simulink model "ES_butterfinger"  (R2017b)
settings: Solver=ode5  StartTime=0.0  StopTime=t_end  FixedStep=dt  RelTol=1e-3
values from neighbouring files (symbols this model uses):
  decimal_year = year + (DOY./365) + (hour./(365.*24)) + (minute./(365.*24.*60)) + (second./(365.*24.*3600))    [Sim_Starter.m]
  DOY = make_doy(year,month,day)    [Sim_Starter.m]    (also in make_doy.m = day + month_doy)
  Ib = [50 0 0; 0 50 0; 0 0 25]    [Sim_Starter.m]
  IC = [r_ECI_i; v_ECI_i; q_i; w_i]    [Sim_Starter.m]
  msc = 50    [Sim_Starter.m]
  sc_area = [1; 1; 1]    [Sim_Starter.m]
  sc_cop = [0; 0; 0]    [Sim_Starter.m]
  year = 2017    [Sim_Starter.m]
undefined symbols (not defined in the file or in its folder): DiscIntNeverNeededParam, Earth, IAU, WGS84
libraries: aerolibtransform2 x3, sharedtransform x3, aerolibatmos2 x1, aerolibgravity2 x1
settings Model: Creator=Mitchel  LastModifiedBy=Mitchel

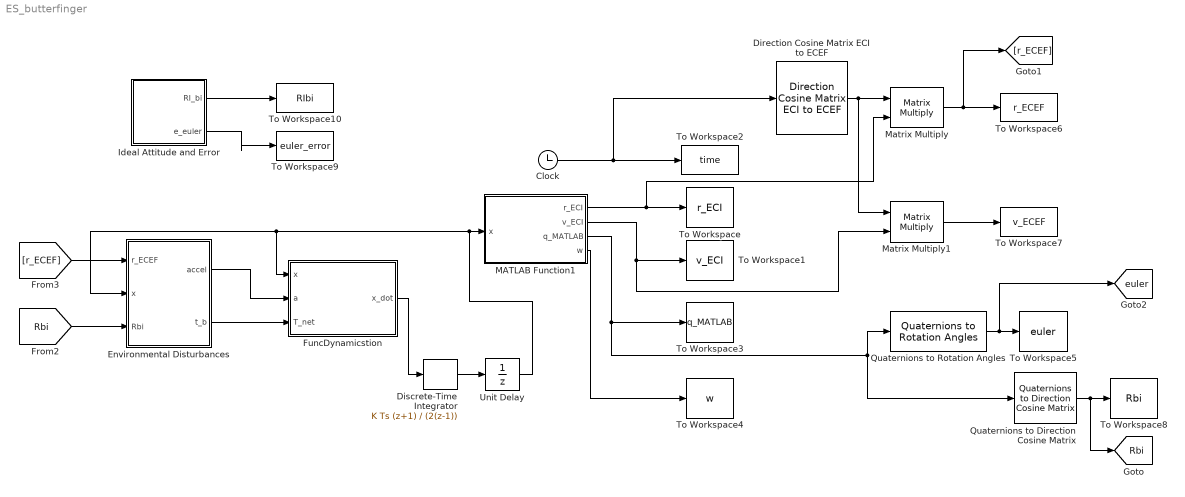
== system ES_butterfinger ==
  Clock : Clock
  Direction Cosine Matrix ECI to ECEF : aerolibtransform2/Direction Cosine Matrix ECI to ECEF  red=IAU-2000/2006  year=year  month=November  day=20  hour=hour  min=minute  sec=second  deltaT=Sec  errorflag=Error  extraparamflag=off
      settings: AttributesFormatString=%<red>  SourceProductName=Aerospace Blockset  SourceProductBaseCode=AE
  Discrete-Time Integrator : DiscreteIntegrator  IntegratorMethod=Integration: Trapezoidal  InitialCondition=IC  InitialConditionSetting=State (most efficient)  SampleTime=-1  ICPrevOutput=DiscIntNeverNeededParam  ICPrevScaledInput=DiscIntNeverNeededParam
  Environmental Disturbances : Subsystem
  FuncDynamicstion : MATLAB Function  TreatAsAtomicUnit=on
  Ideal Attitude and Error : Subsystem
  MATLAB Function1 : MATLAB Function  TreatAsAtomicUnit=on
  Matrix Multiply : Product  Multiplication=Matrix(*)
  Matrix Multiply1 : Product  Multiplication=Matrix(*)
  Quaternions to Direction Cosine Matrix : sharedtransform/Quaternions to  Direction Cosine Matrix
      settings: SourceProductName=Aerospace Blockset  SourceProductBaseCode=AE
  Quaternions to Rotation Angles : sharedtransform/Quaternions to Rotation Angles  rotationOrder=ZYX
      settings: SourceProductBaseCode=AE
  To Workspace : ToWorkspace  VariableName=r_ECI  SampleTime=-1
      settings: Save2DSignal=2-D array (concatenate along first dimension)
  To Workspace1 : ToWorkspace  VariableName=v_ECI  SampleTime=-1
      settings: Save2DSignal=2-D array (concatenate along first dimension)
  To Workspace10 : ToWorkspace  VariableName=RIbi  SampleTime=-1
  To Workspace2 : ToWorkspace  VariableName=time  SampleTime=-1
      settings: Save2DSignal=2-D array (concatenate along first dimension)
  To Workspace3 : ToWorkspace  VariableName=q_MATLAB  SampleTime=-1
      settings: Save2DSignal=2-D array (concatenate along first dimension)
  To Workspace4 : ToWorkspace  VariableName=w  SampleTime=-1
      settings: Save2DSignal=2-D array (concatenate along first dimension)
  To Workspace5 : ToWorkspace  VariableName=euler  SampleTime=-1
      settings: Save2DSignal=2-D array (concatenate along first dimension)
  To Workspace6 : ToWorkspace  VariableName=r_ECEF  SampleTime=-1
      settings: Save2DSignal=2-D array (concatenate along first dimension)
  To Workspace7 : ToWorkspace  VariableName=v_ECEF  SampleTime=-1
      settings: Save2DSignal=2-D array (concatenate along first dimension)
  To Workspace8 : ToWorkspace  VariableName=Rbi  SampleTime=-1
      settings: Save2DSignal=2-D array (concatenate along first dimension)
  To Workspace9 : ToWorkspace  VariableName=euler_error  SampleTime=-1
      settings: Save2DSignal=2-D array (concatenate along first dimension)
  Unit Delay : UnitDelay  InitialCondition=IC  SampleTime=-1
  tag scope: Rbi=global, euler=global
  wires:
  MATLAB Function1/1(r_ECI) -> Matrix Multiply/2, To Workspace/1
  MATLAB Function1/2(v_ECI) -> Matrix Multiply1/2, To Workspace1/1
  Clock/1 -> Direction Cosine Matrix ECI to ECEF/1, To Workspace2/1
  FuncDynamicstion/1(x_dot) -> Discrete-Time Integrator/1
  MATLAB Function1/4(w) -> To Workspace4/1
  Direction Cosine Matrix ECI to ECEF/1 -> Matrix Multiply1/1, Matrix Multiply/1
  Matrix Multiply/1 -> [r_ECEF], To Workspace6/1
  Matrix Multiply1/1 -> To Workspace7/1
  Quaternions to Rotation Angles/1 -> [euler], To Workspace5/1
  Discrete-Time Integrator/1 -> Unit Delay/1
  Unit Delay/1 -> MATLAB Function1/1(x), Environmental Disturbances/2(x), FuncDynamicstion/1(x)
  Quaternions to Direction Cosine Matrix/1 -> [Rbi], To Workspace8/1
  MATLAB Function1/3(q_MATLAB) -> Quaternions to Direction Cosine Matrix/1, Quaternions to Rotation Angles/1, To Workspace3/1
  Environmental Disturbances/2(t_b) -> FuncDynamicstion/3(T_net)
  Environmental Disturbances/1(accel) -> FuncDynamicstion/2(a)
  [Rbi] -> Environmental Disturbances/3(Rbi)
  [r_ECEF] -> Environmental Disturbances/1(r_ECEF)
  Ideal Attitude and Error/1(RI_bi) -> To Workspace10/1
  Ideal Attitude and Error/2(e_euler) -> To Workspace9/1

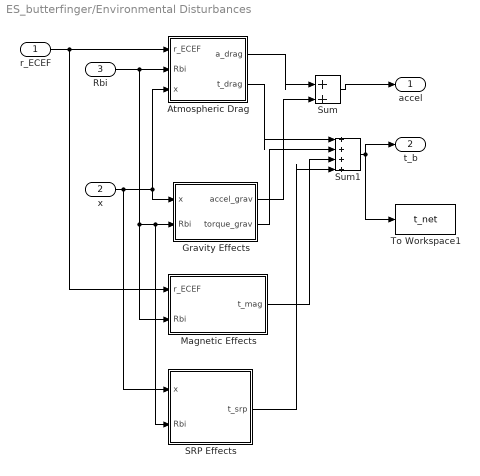
== system ES_butterfinger/Environmental Disturbances ==
  r_ECEF : Inport
  x : Inport  Port=2
  Rbi : Inport  Port=3
  Atmospheric Drag : Subsystem
  "Gravity Effects " : Subsystem
  Magnetic Effects : Subsystem
  "SRP Effects " : Subsystem
  Sum : Sum  Inputs=|++
  Sum1 : Sum  Inputs=|++++
  To Workspace1 : ToWorkspace  VariableName=t_net  SampleTime=-1
  accel : Outport
  t_b : Outport  Port=2
  wires:
  Sum/1 -> accel/1
  Atmospheric Drag/1(a_drag) -> Sum/1
  "Gravity Effects "/1(accel_grav) -> Sum/2
  Sum1/1 -> t_b/1, To Workspace1/1
  Atmospheric Drag/2(t_drag) -> Sum1/1
  r_ECEF/1 -> Magnetic Effects/1(r_ECEF), Atmospheric Drag/1(r_ECEF)
  Rbi/1 -> "SRP Effects "/2(Rbi), "Gravity Effects "/2(Rbi), Magnetic Effects/2(Rbi), Atmospheric Drag/2(Rbi)
  "Gravity Effects "/2(torque_grav) -> Sum1/2
  Magnetic Effects/1(t_mag) -> Sum1/3
  x/1 -> "SRP Effects "/1(x), Atmospheric Drag/3("x "), "Gravity Effects "/1(x)
  "SRP Effects "/1("t_srp ") -> Sum1/4

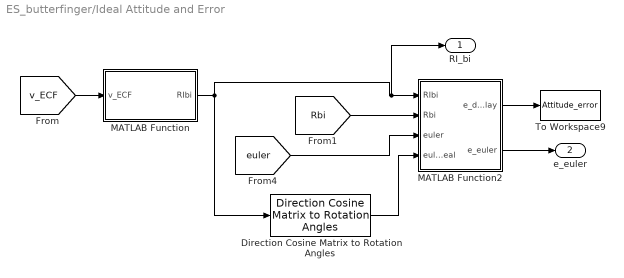
== system ES_butterfinger/Ideal Attitude and Error ==
  Direction Cosine Matrix to Rotation Angles : sharedtransform/Direction Cosine Matrix to Rotation Angles  rotationOrder=ZYX
      settings: SourceProductName=Aerospace Blockset  SourceProductBaseCode=AE
  MATLAB Function : MATLAB Function  TreatAsAtomicUnit=on
  MATLAB Function2 : MATLAB Function  TreatAsAtomicUnit=on
  To Workspace9 : ToWorkspace  VariableName=Attitude_error  SampleTime=-1
      settings: Save2DSignal=2-D array (concatenate along first dimension)
  RI_bi : Outport
  e_euler : Outport  Port=2
  wires:
  MATLAB Function2/1(e_display) -> To Workspace9/1
  [v_ECF] -> MATLAB Function/1(v_ECF)
  MATLAB Function2/2(e_euler) -> e_euler/1
  [euler] -> MATLAB Function2/3(euler)
  Direction Cosine Matrix to Rotation Angles/1 -> MATLAB Function2/4(euler_ideal)
  MATLAB Function/1(RIbi) -> Direction Cosine Matrix to Rotation Angles/1, RI_bi/1, MATLAB Function2/1(RIbi)
  [Rbi] -> MATLAB Function2/2(Rbi)

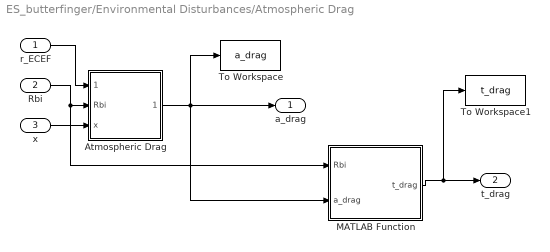
== system ES_butterfinger/Environmental Disturbances/Atmospheric Drag ==
  r_ECEF : Inport
  Rbi : Inport  Port=2
  "x " : Inport  Port=3
  Atmospheric Drag : Subsystem
  MATLAB Function : MATLAB Function  TreatAsAtomicUnit=on
  To Workspace : ToWorkspace  VariableName=a_drag  SampleTime=-1
  To Workspace1 : ToWorkspace  VariableName=t_drag  SampleTime=-1
  a_drag : Outport
  t_drag : Outport  Port=2
  wires:
  MATLAB Function/1(t_drag) -> To Workspace1/1, t_drag/1
  "x "/1 -> Atmospheric Drag/3(x)
  Rbi/1 -> MATLAB Function/1(Rbi), Atmospheric Drag/2(Rbi)
  r_ECEF/1 -> Atmospheric Drag/1(r_ECEF)
  Atmospheric Drag/1(a_drag) -> MATLAB Function/2(a_drag), To Workspace/1, a_drag/1

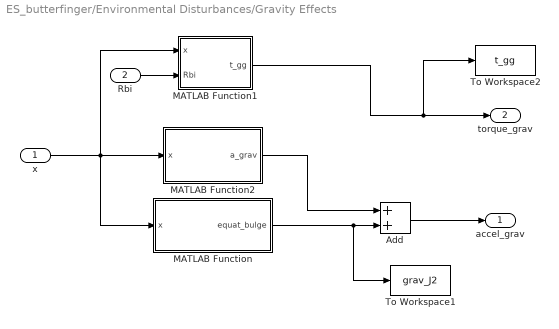
== system ES_butterfinger/Environmental Disturbances/Gravity Effects  ==
  x : Inport
  Rbi : Inport  Port=2
  Add : Sum
  MATLAB Function : MATLAB Function  TreatAsAtomicUnit=on
  MATLAB Function1 : MATLAB Function  TreatAsAtomicUnit=on
  MATLAB Function2 : MATLAB Function  TreatAsAtomicUnit=on
  To Workspace1 : ToWorkspace  VariableName=grav_J2  SampleTime=-1
  To Workspace2 : ToWorkspace  VariableName=t_gg  SampleTime=-1
  accel_grav : Outport
  torque_grav : Outport  Port=2
  wires:
  MATLAB Function2/1(a_grav) -> Add/1
  x/1 -> MATLAB Function1/1(x), MATLAB Function/1(x), MATLAB Function2/1(x)
  MATLAB Function/1(equat_bulge) -> To Workspace1/1, Add/2
  Add/1 -> accel_grav/1
  Rbi/1 -> MATLAB Function1/2(Rbi)
  MATLAB Function1/1(t_gg) -> To Workspace2/1, torque_grav/1

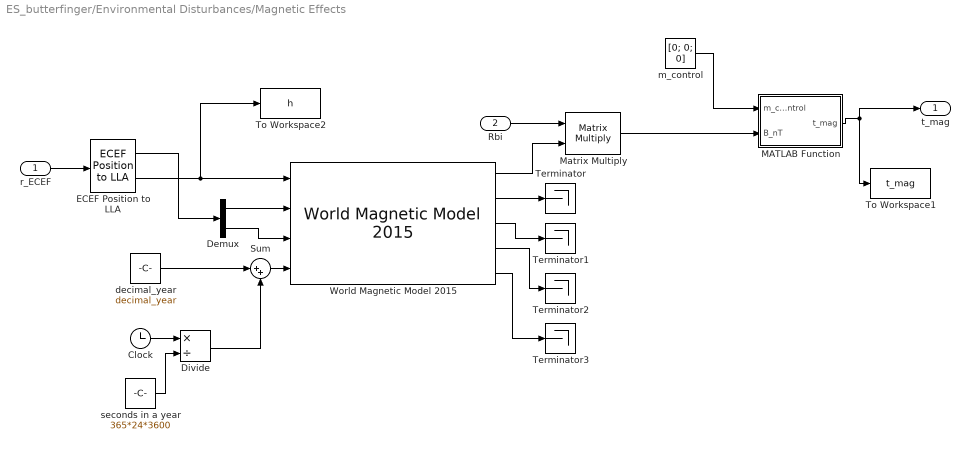
== system ES_butterfinger/Environmental Disturbances/Magnetic Effects ==
  r_ECEF : Inport
  Rbi : Inport  Port=2
  Clock : Clock
  Demux : Demux  Outputs=2
  Divide : Product  Inputs=*/
  ECEF Position to LLA : aerolibtransform2/ECEF Position to LLA  units=Metric (MKS)  ptype=Earth (WGS84)  F=1/298.257223563  R=6378137
      settings: SourceProductName=Aerospace Blockset  SourceProductBaseCode=AE
  MATLAB Function : MATLAB Function  TreatAsAtomicUnit=on
  Matrix Multiply : Product  Multiplication=Matrix(*)
  Sum : Sum  Inputs=|++
  Terminator{,1..3} (4 alike) : Terminator
  To Workspace1 : ToWorkspace  VariableName=t_mag  SampleTime=-1
      settings: Save2DSignal=2-D array (concatenate along first dimension)
  To Workspace2 : ToWorkspace  VariableName=h  SampleTime=-1
  World Magnetic Model 2015 : aerolibgravity2/World Magnetic Model 2015  units=Metric (MKS)  time_in=on  month=November  day=20  year=2015  action=Error  h_out=on  dec_out=on  inc_out=on  ti_out=on
      settings: SourceProductName=Aerospace Blockset  SourceProductBaseCode=AE
  "decimal_year " : Constant  Value=decimal_year
  m_control : Constant  Value=[0; 0; 0]
  seconds in a year : Constant  Value=365*24*3600
  t_mag : Outport
  wires:
  World Magnetic Model 2015/3 -> Terminator1/1
  World Magnetic Model 2015/4 -> Terminator2/1
  World Magnetic Model 2015/5 -> Terminator3/1
  MATLAB Function/1(t_mag) -> t_mag/1, To Workspace1/1
  World Magnetic Model 2015/2 -> Terminator/1
  r_ECEF/1 -> ECEF Position to LLA/1
  Demux/1 -> World Magnetic Model 2015/2
  Demux/2 -> World Magnetic Model 2015/3
  ECEF Position to LLA/1 -> Demux/1
  ECEF Position to LLA/2 -> To Workspace2/1, World Magnetic Model 2015/1
  m_control/1 -> MATLAB Function/1(m_control)
  seconds in a year/1 -> Divide/2
  Clock/1 -> Divide/1
  "decimal_year "/1 -> Sum/1
  Divide/1 -> Sum/2
  Sum/1 -> World Magnetic Model 2015/4
  Rbi/1 -> Matrix Multiply/1
  World Magnetic Model 2015/1 -> Matrix Multiply/2
  Matrix Multiply/1 -> MATLAB Function/2(B_nT)

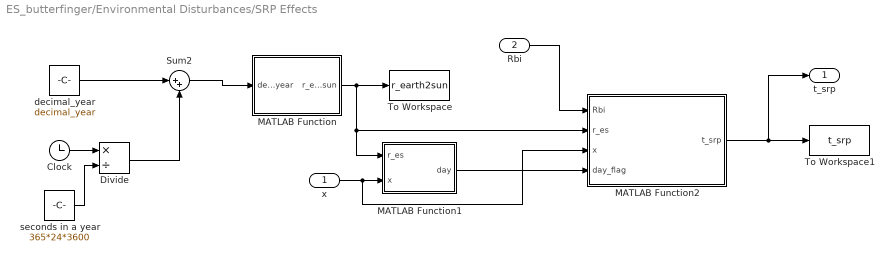
== system ES_butterfinger/Environmental Disturbances/SRP Effects  ==
  x : Inport
  Rbi : Inport  Port=2
  Clock : Clock
  Divide : Product  Inputs=*/
  MATLAB Function : MATLAB Function  TreatAsAtomicUnit=on
  MATLAB Function1 : MATLAB Function  TreatAsAtomicUnit=on
  MATLAB Function2 : MATLAB Function  TreatAsAtomicUnit=on
  Sum2 : Sum  Inputs=|++
  To Workspace : ToWorkspace  VariableName=r_earth2sun  SampleTime=-1
  To Workspace1 : ToWorkspace  VariableName=t_srp  SampleTime=-1
  "decimal_year " : Constant  Value=decimal_year
  seconds in a year : Constant  Value=365*24*3600
  "t_srp " : Outport
  wires:
  Divide/1 -> Sum2/2
  Clock/1 -> Divide/1
  seconds in a year/1 -> Divide/2
  "decimal_year "/1 -> Sum2/1
  Sum2/1 -> MATLAB Function/1(decimal_year)
  MATLAB Function/1(r_earth2sun) -> MATLAB Function2/2(r_es), MATLAB Function1/1(r_es), To Workspace/1
  x/1 -> MATLAB Function2/3(x), MATLAB Function1/2(x)
  MATLAB Function1/1(day) -> MATLAB Function2/4(day_flag)
  Rbi/1 -> MATLAB Function2/1(Rbi)
  MATLAB Function2/1(t_srp) -> "t_srp "/1, To Workspace1/1

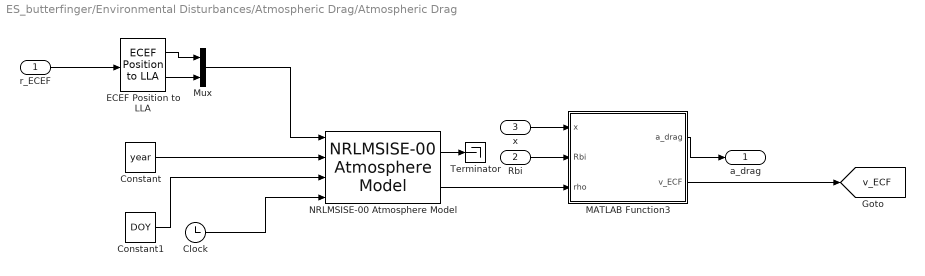
== system ES_butterfinger/Environmental Disturbances/Atmospheric Drag/Atmospheric Drag ==
  r_ECEF : Inport
  Rbi : Inport  Port=2
  x : Inport  Port=3
  Clock : Clock
  Constant : Constant  Value=year
  Constant1 : Constant  Value=DOY
  ECEF Position to LLA : aerolibtransform2/ECEF Position to LLA  units=Metric (MKS)  ptype=Earth (WGS84)  F=1/298.257223563  R=6378137
      settings: SourceProductName=Aerospace Blockset  SourceProductBaseCode=AE
  MATLAB Function3 : MATLAB Function  TreatAsAtomicUnit=on
  Mux : Mux  Inputs=2
  NRLMSISE-00 Atmosphere Model : aerolibatmos2/NRLMSISE-00 Atmosphere Model  units=Metric (MKS)  lst_input=off  flux_ap_input=off  flags_input=Internal  flags=ones(1,23)  oxygen_in=off  action=Warning
      settings: SourceProductName=Aerospace Blockset  SourceProductBaseCode=AE
  Terminator : Terminator
  a_drag : Outport
  tag scope: v_ECF=global
  wires:
  Rbi/1 -> MATLAB Function3/2(Rbi)
  MATLAB Function3/1(a_drag) -> a_drag/1
  r_ECEF/1 -> ECEF Position to LLA/1
  NRLMSISE-00 Atmosphere Model/1 -> Terminator/1
  Constant/1 -> NRLMSISE-00 Atmosphere Model/2
  Clock/1 -> NRLMSISE-00 Atmosphere Model/4
  Constant1/1 -> NRLMSISE-00 Atmosphere Model/3
  ECEF Position to LLA/2 -> Mux/2
  ECEF Position to LLA/1 -> Mux/1
  Mux/1 -> NRLMSISE-00 Atmosphere Model/1
  NRLMSISE-00 Atmosphere Model/2 -> MATLAB Function3/3(rho)
  x/1 -> MATLAB Function3/1(x)
  MATLAB Function3/2(v_ECF) -> [v_ECF]

== matlab function ES_butterfinger/MATLAB Function1 ==
  data: x input; r_ECI output; v_ECI output; q_MATLAB output; w output
function [r_ECI,v_ECI,q_MATLAB,w] = analysis_demux(x)

r_ECI = zeros(3,1);
r_ECI(1,1) = x(1,1);
r_ECI(2,1) = x(2,1);
r_ECI(3,1) = x(3,1);

v_ECI = zeros(3,1);
v_ECI(1,1) = x(4,1);
v_ECI(2,1) = x(5,1);
v_ECI(3,1) = x(6,1);

q_MATLAB = zeros(4,1); %output quaternion in MATLAB notation, not Dogan notation.
q_MATLAB(2,1) = x(7,1);
q_MATLAB(3,1) = x(8,1);
q_MATLAB(4,1) = x(9,1);
q_MATLAB(1,1) = x(10,1);

w = zeros(3,1);
w(1,1) = x(11,1);
w(2,1) = x(12,1);
w(3,1) = x(13,1);
end

== matlab function ES_butterfinger/FuncDynamicstion ==
  data: x input; x_dot output; a input; T_net input; Ib parameter
function x_dot  = state_space(x,a, T_net,Ib)

%1. Translational State Space Equations
%x: [rx; ry; rz; vx; vy; vz; q1; q2; q3; q4; wx; wy; wz]
%NOTE: quaternion uses Dogan Notation.

v = [x(4,1); x(5,1); x(6,1)];

%2. Rotational State Space Equations
q_top = [x(7,1); x(8,1); x(9,1)];
q_bot = x(10,1);
w = [x(11,1); x(12,1); x(13,1)];

S_w = [0 w(3,1) -w(2,1); -w(3,1) 0 w(1,1); w(2,1) -w(1,1) 0];

%q_dot equations - rotational kinematics of a quaternion:
q_dot_top = (1./2).*(S_w*q_top) + (1./2).*q_bot*w;
q_dot_bot = -(1./2).*transpose(w)*q_top;

%angular accleration equations - equations of motion:
w_dot = inv(Ib)*(T_net + -S_w*(Ib*w));

x_dot = [v; a; q_dot_top; q_dot_bot; w_dot];

== matlab function ES_butterfinger/Environmental Disturbances/Gravity Effects /MATLAB Function2 ==
  data: a_grav output; x input
function a_grav = Kep_Grav(x)
% "inverse square" gravity model
r_ECI = [x(1,1); x(2,1); x(3,1)];

mu_e = 3.986004418E+14;
a_grav = ((-1.*mu_e)./(norm(r_ECI).^3)).*(r_ECI);

== matlab function ES_butterfinger/Environmental Disturbances/Atmospheric Drag/Atmospheric Drag/MATLAB Function3 ==
  data: x input; Rbi input; a_drag output; rho input; msc parameter; sc_area parameter; v_ECF output
function [a_drag,v_ECF] = fcn(x,Rbi, rho, msc, sc_area)

%atmospheric drag solver - from Vallado
%M. McDonald 10/15/17

r_ECI = [x(1,1); x(2,1); x(3,1)];
v_ECI = [x(4,1); x(5,1); x(6,1)];

w_e = [0; 0; (7.2921150E-5)];
S_w = [0 w_e(3,1) -w_e(2,1); -w_e(3,1) 0 w_e(1,1); w_e(2,1) -w_e(1,1) 0];

v_ECF = v_ECI + S_w*r_ECI;


Cd = 2.0; %Wertz

%Figure out Av:
Av = norm(transpose(transpose(Rbi)*sc_area)*(v_ECF./norm(v_ECF)));

%determine a_drag_ecef
a_drag = (-1./2).*Cd.*rho(6).*(Av./msc).*(norm(v_ECF)).*(v_ECF);

== matlab function ES_butterfinger/Environmental Disturbances/Gravity Effects /MATLAB Function ==
  data: x input; equat_bulge output
function equat_bulge = grav_J2(x)
r_ECI = [x(1,1); x(2,1); x(3,1)];
r = norm(r_ECI);
%setup constants
mu_e = 3.986004418E+14;
re = 6378137; %radius of the earth - meters
J2 = 1.0826.*(10.^-3);

x_dd = ((mu_e.*r_ECI(1,1))./(r.^3)).*J2.*(3./2).*((re./r).^2).*(5.*((r_ECI(3,1).^2)./(r.^2))-1);
y_dd = ((mu_e.*r_ECI(2,1))./(r.^3)).*J2.*(3./2).*((re./r).^2).*(5.*((r_ECI(3,1).^2)./(r.^2))-1);
z_dd = ((-mu_e.*r_ECI(3,1))./(r.^3)).*J2.*(3./2).*((re./r).^3).*(3-5.*((r_ECI(3,1).^2)./(r.^2)));

equat_bulge = [x_dd; y_dd; z_dd];

== matlab function ES_butterfinger/Environmental Disturbances/Atmospheric Drag/MATLAB Function ==
  data: Rbi input; t_drag output; a_drag input; sc_cop parameter; msc parameter
function t_drag = fcn(Rbi,a_drag,sc_cop, msc)

S_sc_cop = [0 sc_cop(3,1) -sc_cop(2,1); -sc_cop(3,1) 0 sc_cop(1,1); sc_cop(2,1) -sc_cop(1,1) 0];

t_drag = -S_sc_cop*(Rbi*(msc.*a_drag));

== matlab function ES_butterfinger/Environmental Disturbances/Gravity Effects /MATLAB Function1 ==
  data: t_gg output; x input; Rbi input; msc parameter; Ib parameter
function t_gg = fcn(x,Rbi, msc, Ib)
r_ECI = [x(1,1); x(2,1); x(3,1)];

mu_e = 3.986004418E+14;
r = norm(r_ECI);

rb = Rbi*r_ECI;

S_rb = [0 rb(3,1) -rb(2,1); -rb(3,1) 0 rb(1,1); rb(2,1) -rb(1,1) 0];

t_gg = ((3.*msc.*mu_e)./(r.^5)).*(-S_rb*Ib*rb);

== matlab function ES_butterfinger/Environmental Disturbances/Magnetic Effects/MATLAB Function ==
  data: t_mag output size=3; m_control input; B_nT input; m_bus parameter
function t_mag = fcn(m_control, B_nT, m_bus)

m = m_bus + m_control;
S_m = [0 m(3,1) -m(2,1); -m(3,1) 0 m(1,1); m(2,1) -m(1,1) 0];

B = (B_nT.*(1.*(10.^-9)));
t_mag = -S_m*B;

== matlab function ES_butterfinger/Environmental Disturbances/SRP Effects /MATLAB Function ==
  data: decimal_year input; r_earth2sun output
function r_earth2sun = kepler2cart(decimal_year)

%2-Body Earth-Sun Orbital Parameters:
%From JPL (https://nssdc.gsfc.nasa.gov/planetary/factsheet/earthfact.html)
a = (149.60).*(10.^6).*(10.^3); %semimajor axis, m
e = 0.0167; %Orbit Eccentricity
i = 0;
omega = deg2rad(102.94719); %long. of perihelion
OMEGA = deg2rad(174.9); %long. of ascending node

year_int = floor(decimal_year);

SOP = 1;
%E = ((decimal_year - year_int)./(SOP)).*(2.*pi); %eccentric anomaly, in radians
%IMPORTANT NOTE: an approximation is made that E = M since eccentricity is
%small.
% vern_eq = [2017 79 10 29 00]; %closest vernal equinox date.
% vern_eq_y = vern_eq(1,1) + (vern_eq(1,2)./365) + (vern_eq(1,3)./(365.*24)) + (vern_eq(1,4)./(365.*24.*60)) + (vern_eq(1,5)./(365.*24.*3600));

%dt_y = (decimal_year - vern_eq_y) - floor((decimal_year - vern_eq_y));
dt_y = decimal_year - floor(decimal_year);
E = ((dt_y).*(2.*pi)); %eccentric anomaly, in radians.

phi = acos((cos(E) - e)./(1 - e.*cos(E)));


p = a.*(1 - (e.^2));
r = (p./(1 + e.*cos(phi)));

% p_vec = [(cos(OMEGA).*cos(omega) - sin(OMEGA).*sin(omega).*cos(i)); ...
%     (-cos(OMEGA).*sin(omega) - sin(OMEGA).*sin(omega).*cos(i)); ...
%     sin(OMEGA).*sin(i)];
% 
% q_vec = [(sin(OMEGA).*cos(omega) + cos(OMEGA).*sin(omega).*cos(i)); ...
%     (-sin(OMEGA).*sin(omega) + cos(OMEGA).*cos(omega).*cos(i)); ...
%     -cos(OMEGA).*sin(i)];

p_vec = [(cos(OMEGA).*cos(omega) - sin(OMEGA).*sin(omega).*cos(i)); ...
    (sin(OMEGA).*cos(omega) + sin(OMEGA).*sin(omega).*cos(i)); ...
    sin(omega).*sin(i)];

q_vec = [(-cos(OMEGA).*sin(omega) - sin(OMEGA).*cos(omega).*cos(i)); ...
    (-sin(OMEGA).*sin(omega) + cos(OMEGA).*cos(omega).*cos(i)); ...
    cos(omega).*sin(i)];


%p_vec.*cos(phi) + q_vec.*sin(phi)
r_earth2sun_e = r.*(p_vec.*cos(phi) + q_vec.*sin(phi)); %location of earth w/respect to sun centered ecliptic frame


theta = deg2rad(23.4);
RJe = [1 0 0;...
    0 cos(theta) -sin(theta); ...
    0 sin(theta) cos(theta)]; %rotation from Ecliptic frame to J2000.

r_earth2sun = RJe*(-r_earth2sun_e); %position of sun relative to earth in ECI.
%r_sun2earth = r_earth2sun_e;
end

== matlab function ES_butterfinger/Environmental Disturbances/SRP Effects /MATLAB Function1 ==
  data: r_es input; day output; x input
function day = day_flag(r_es, x)

%A very rough approximation to account for night/day effects.
%Since this sim is for orbits >600km in altitude, it is assumed that
%'night/day' transition occurs when the vehicle is at the solar horizon.

r_ECI = [x(1,1); x(2,1); x(3,1)];

theta = acos((dot(r_es,r_ECI))./(norm(r_es).*norm(r_ECI)));


if cos(theta) < 0
    day = 0; %'night' time
else
    day = 1; %'day' flag

end

== matlab function ES_butterfinger/Environmental Disturbances/SRP Effects /MATLAB Function2 ==
  data: Rbi input; t_srp output; r_es input; x input; day_flag input; sc_area parameter; sc_cop parameter
function t_srp = t_solar(Rbi,r_es, x, day_flag, sc_area, sc_cop)
%from: http://ccar.colorado.edu/ASEN5050/ASEN5050/Lectures_files/lecture22.pdf
%From Jeffery Parker Lecture U of Boulder.
r_ECI = [x(1,1); x(2,1); x(3,1)];

r_sat = r_es - r_ECI; %vector from satellite to sun in ECI (meters).
%convert to body frame:
r_sat_b = Rbi*r_sat;

%Figure out Av:
Av = norm(transpose(transpose(Rbi)*sc_area)*(r_sat_b./norm(r_sat_b)));

psr = 4.57E-6; %W*s/m^3
cr = 0.6; %satellite reflectivity

F_SRP = -((psr.*cr.*Av.*(r_sat_b))./(abs(r_sat_b)));
t_srp = day_flag.*cross(sc_cop,F_SRP);

== matlab function ES_butterfinger/Ideal Attitude and Error/MATLAB Function ==
  data: v_ECF input; RIbi output; Rab parameter
function RIbi  = IdealAtt(v_ECF, Rab)

    %Determine rotation from inertial ECI to v_ECF in axis-angle
    %coordinates:
    
    x_ECI = [1 0 0];
    
    phi = acos((dot(v_ECF,x_ECI))./(norm(v_ECF).*norm(x_ECI)));
    
    v_ECF_n = v_ECF./norm(v_ECF);
    c = cross(x_ECI,v_ECF_n)';
    
    %Converting from axis-angle to Rotation Matrix:
    S_c = [0 c(3,1) -c(2,1);
        -c(3,1) 0 c(1,1);
        c(2,1) -c(1,1) 0];
    
    S_c_phi = S_c.*phi;
    Rai = expm(S_c_phi);
    
    %Find "Ideal" Attitude for Maximum Drag:
    RIbi = transpose(Rab)*Rai;
end

== matlab function ES_butterfinger/Ideal Attitude and Error/MATLAB Function2 ==
  data: RIbi input; e_display output; Rbi input; e_euler output; euler input; euler_ideal input
function [e_display,e_euler] = AttError(RIbi, Rbi,euler, euler_ideal)
%Determines error angle between Ideal and Actual Attitude.
%From Mortari AERO-423 Notes:

%Determine overall attitude error (in degrees)
T = RIbi;
C = Rbi;

cos_e = (.5).*(trace(T*transpose(C)) -1 );
%error angle is in degrees.
e_display = acosd(cos_e);

%Determine Controller Attitude Error in Euler Angles, radians
e_euler = euler - euler_ideal;

end
